simulink library "hcu_lib"  (R2021b)
settings: Solver=VariableStepAuto  StartTime=0.0  StopTime=10.0  RelTol=1e-3
undefined symbols (not defined in the file): ENUM_FAULTSTATE_FAIL, ENUM_FAULTSTATE_INDETERMINATE, ENUM_FAULTSTATE_PASS, EPSILON, FALSE, KPH2MPH, KPH2MPS, KXX2XX, MPH2KPH, MPS2KPH, ONE_INT16, ONE_INT32, RADPS2RPM, RPM2RADPS, slcm, TRUE, UNDEFINED_VALUE, XX2KXX, ZERO_FLOAT, ZERO_INT, ZERO_INT16, ZERO_INT32
libraries: $bdroot x31, simulink x10, afl x1
(part 1 of 3)
settings Model: Creator=12018  LastModifiedBy=FVT23010
settings SolverCC: AlgebraicLoopSolver=TrustRegion
settings DataIOCC: LimitDataPoints=on  SaveFormat=Array  SignalLoggingSaveFormat=ModelDataLogs  ReturnWorkspaceOutputs=off
settings OptimizationCC: BlockReduction=off  BooleanDataType=off  LifeSpan=inf
settings DebuggingCC: SaveWithParameterizedLinksMsg=none  UnderspecifiedInitializationDetection=Classic  MergeDetectMultiDrivingBlocksExec=none  SignalResolutionControl=TryResolveAllWithWarning  AllowSymbolicDim=off  SFUnexpectedBacktrackingDiag=warning  SFNoUnconditionalDefaultTransitionDiag=warning  SFExecutionAtInitializationDiag=none  SFMachineParentedDataDiag=warning  ArithmeticOperatorsInVariantConditions=warning
settings HardwareCC: TargetUnknown=on
settings ModelReferenceCC: PropagateSignalLabelsOutOfModel=off
settings SFSimCC: SimUseLocalCustomCode=off  CustomCodeUndefinedFunction=UseInterfaceOnly
settings RTWCC: RTWUseLocalCustomCode=off
settings CodeAppCC: StateflowObjectComments=on
settings GRTTargetCC: TargetLangStandard=C89/C90 (ANSI)
settings ConfigComp: CovMetricSettings=dw  CovSaveCumulativeToWorkspaceVar=on  CovSaveSingleToWorkspaceVar=on  CovExternalEMLEnable=off

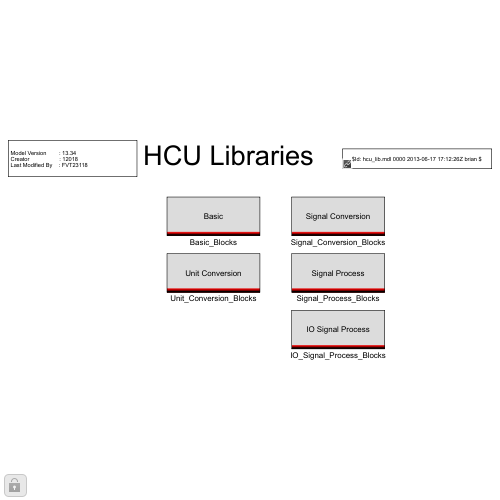
[thumbnail: Simulink's stored preview of the top-level diagram]
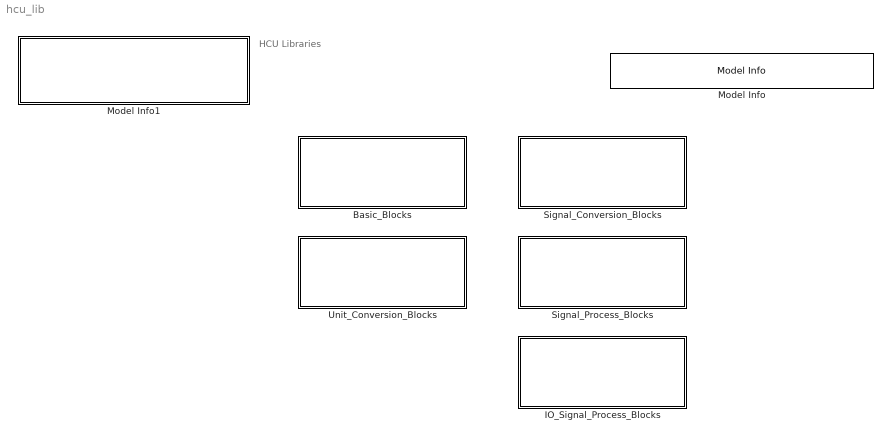
== system hcu_lib ==
  note: HCU Libraries
  Basic_Blocks : Subsystem
      mask Display:
      | patch([0 0 1 1], [0 1 1 0], [220/255 220/255 220/255]);
      | patch([0 0 1 1], [0 0.075 0.075 0], [230/255 0/255 0/255]);
      | patch([0 0 1 1], [0.025 0.05 0.05 0.025], [150/255 0/255 0/255]);
      | patch([0 0 1 1], [0 0.025 0.025 0], [0/255 0/255 0/255]);
      | 
      | disp('Basic')
  IO_Signal_Process_Blocks : Subsystem
      mask Display:
      | patch([0 0 1 1], [0 1 1 0], [220/255 220/255 220/255]);
      | patch([0 0 1 1], [0 0.075 0.075 0], [230/255 0/255 0/255]);
      | patch([0 0 1 1], [0.025 0.05 0.05 0.025], [150/255 0/255 0/255]);
      | patch([0 0 1 1], [0 0.025 0.025 0], [0/255 0/255 0/255]);
      | 
      | disp('IO Signal Process')
  Model Info : simulink/Model-Wide Utilities/Model Info  Frame=on  DisplayStringWithTags=$Id: hcu_lib.mdl 0000 2013-06-17 17:12:26Z brian $  HorizontalTextAlignment=Center  LeftAlignmentValue=0.5
  Model Info1 : Subsystem  LoadFcn=slcm LoadBlock;  InitFcn=slcm('UpdateAllCMBlocksInThisModelInit')  mask(CMBlock){InitialSaveTempField=, InitialBlockCM=, BlockCM=None, Frame=on, SaveTempField=, DisplayStringWithTags=|, MaskDisplayString=Model Version        : 13.85\nCreator                   : 12018\nLast Modified By    : FVT23010, HorizontalTextAlignment=Left, LeftAlignmentValue=0.02, SourceBlockDiagram=hcu_lib, TagMaxNumber=20, CMTag1=, CMTag2=, CMTag3=, CMTag4=, CMTag5=, CMTag6=, CMTag7=, CMTag8=, CMTag9=, CMTag10=, CMTag11=, CMTag12=, CMTag13=, CMTag14=, CMTag15=, CMTag16=, CMTag17=, CMTag18=, CMTag19=, CMTag20=}
      mask DisplayStringWithTags=|
      | Model Version        : %<ModelVersion>
      | Creator                   : %<Creator>
      | Last Modified By    : %<LastModifiedBy>
      mask help: This block allows revision control information to be displayed within the model.
      settings: CopyFcn=slcm CopyBlock;  DeleteFcn=slcm Cancel;  PostSaveFcn=slcm('UpdateAllCMBlocksInThisModel')  NameChangeFcn=slcm Rename;  OpenFcn=slcm
      mask Display: text(str2num(LeftAlignmentValue), 0.5, MaskDisplayString, 'HorizontalAlignment', HorizontalTextAlignment)
  Signal_Conversion_Blocks : Subsystem
      mask Display:
      | patch([0 0 1 1], [0 1 1 0], [220/255 220/255 220/255]);
      | patch([0 0 1 1], [0 0.075 0.075 0], [230/255 0/255 0/255]);
      | patch([0 0 1 1], [0.025 0.05 0.05 0.025], [150/255 0/255 0/255]);
      | patch([0 0 1 1], [0 0.025 0.025 0], [0/255 0/255 0/255]);
      | 
      | disp('Signal Conversion')
  Signal_Process_Blocks : Subsystem
      mask Display:
      | patch([0 0 1 1], [0 1 1 0], [220/255 220/255 220/255]);
      | patch([0 0 1 1], [0 0.075 0.075 0], [230/255 0/255 0/255]);
      | patch([0 0 1 1], [0.025 0.05 0.05 0.025], [150/255 0/255 0/255]);
      | patch([0 0 1 1], [0 0.025 0.025 0], [0/255 0/255 0/255]);
      | 
      | disp('Signal Process')
  Unit_Conversion_Blocks : Subsystem
      mask Display:
      | patch([0 0 1 1], [0 1 1 0], [220/255 220/255 220/255]);
      | patch([0 0 1 1], [0 0.075 0.075 0], [230/255 0/255 0/255]);
      | patch([0 0 1 1], [0.025 0.05 0.05 0.025], [150/255 0/255 0/255]);
      | patch([0 0 1 1], [0 0.025 0.025 0], [0/255 0/255 0/255]);
      | 
      | disp('Unit Conversion')

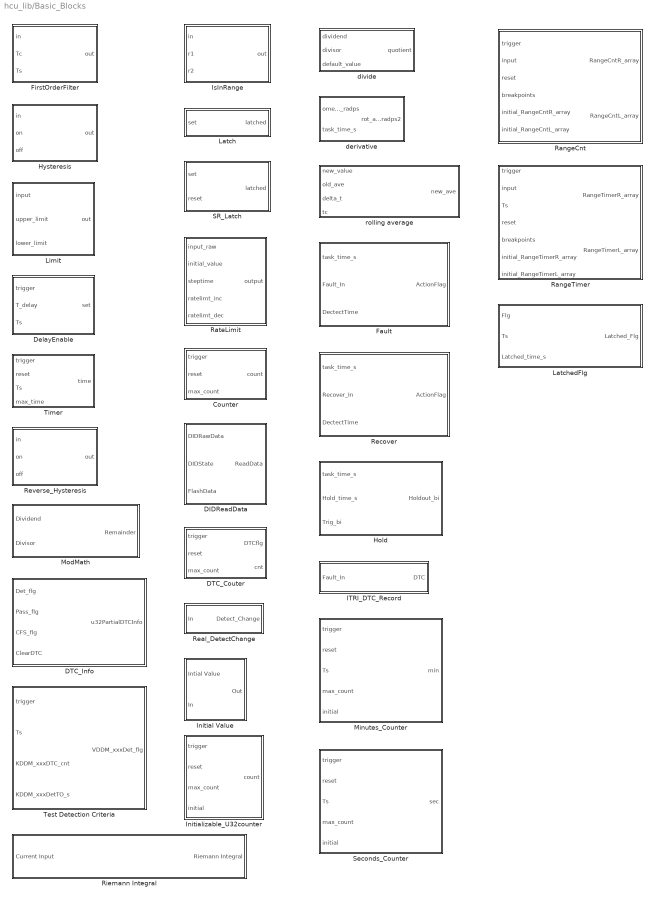
== system hcu_lib/Basic_Blocks ==
  Counter : Subsystem  mask(Count){}
      mask help: Counter function.
  DIDReadData : Subsystem  mask(Count){}
      mask help: Counter function.
  DTC_Couter : Subsystem  mask(Count){}
      mask help: Counter function.
  DTC_Info : Subsystem
  DelayEnable : Subsystem  mask(DelayEnable){}
      mask help: Delay enable funcion.
  Fault : Subsystem
  FirstOrderFilter : Subsystem  TreatAsAtomicUnit=on  RTWFileName=HCU_LIB  mask(FirstOrderFilter){}
      mask help: First order Filter.
      settings: RTWSystemCode=Inline  RTWFileNameOpts=User specified
  Hold : Subsystem
  Hysteresis : Subsystem  RTWFileName=HCU_LIB  mask(Hysteresis){}
      mask help: Hysteresis funcion.
      settings: RTWFileNameOpts=User specified
  ITRI_DTC_Record : Subsystem
  Initial Value : Subsystem  mask(Count){}
      mask help: Counter function.
  Initializable_U32counter : Subsystem  mask(Count){}
      mask help: Counter function.
  IsInRange : Subsystem  RTWFileName=HCU_LIB  mask(IsInRange){}
      mask help: Check the value range.
      settings: RTWFileNameOpts=User specified
  Latch : Subsystem  mask(Latch){}
      mask help: Latch function.
  LatchedFlg : Subsystem  mask(Latched Flg){}
      mask help: Latch flg function.
  Limit : Subsystem  RTWFileName=HCU_LIB  mask(Limit){}
      mask help: Limit funcion.
      settings: RTWFileNameOpts=User specified
  Minutes_Counter : Subsystem  mask(Min Count){}
      mask help: Minutes Counter.
  ModMath : Subsystem  mask(Count){}
      mask help: Counter function.
      mask Display:
      | fprintf('ModMath');
      | port_label('output', 1, 'Remainder');
      | port_label('input', 1, 'Dividend');
      | port_label('input', 2, 'Divisor');
  RangeCnt : Subsystem  mask(RangeCnt){}
      mask help: Range Counter.
  RangeTimer : Subsystem  mask(RangeTimer){}
      mask help: Range Timer (sec).
  RateLimit : Subsystem  RTWFileName=HCU_LIB  mask(RateLimit){}
      mask help: Rate limit function.
      settings: RTWFileNameOpts=User specified
  Real_DetectChange : Subsystem  mask(Count){}
      mask help: Counter function.
  Recover : Subsystem
  Reverse_Hysteresis : Subsystem  RTWFileName=HCU_LIB  mask(Hysteresis){}
      mask help: Hysteresis funcion.
      settings: RTWFileNameOpts=User specified
  Riemann Integral : Subsystem  mask(Riemann Integral){Ts=0.005, Total_T=1}
      mask prompts: Ts "Ts (s)"; Total_T "Total Time Interval (s)"
      mask help: Riemann Integral.
      mask Display:
      | fprintf('Ts (s): %4.3f \n Total Time Interval (s): %4.3f', Ts, Total_T);
      | 
      | port_label('input', 1, 'Current Input');
      | 
      | port_label('output', 1, ' Riemann Integral');
  SR_Latch : Subsystem  mask(SR_Latch){}
      mask help: SR latch function.
  Seconds_Counter : Subsystem  mask(Sec Count){}
      mask help: Seconds Counter.
  Test Detection Criteria : Subsystem
  Timer : Subsystem  mask(Timer){}
      mask help: Timer funcion.
  derivative : Subsystem  mask(Derative Block){}
      mask help: Simplified Derivative Calculation
      mask Display: disp(['Derivative'])
  divide : Subsystem  RTWFcnName=plaus_check  mask(divide){}
      mask help: Performs a division operation. If the divisor is found to be between -0.00001 and +0.00001 then a failsafe value is passed to the output.
      settings: RTWFcnNameOpts=User specified
      mask Display: disp('Divide');
  rolling average : Subsystem  RTWFcnName=rolav_tc  RTWFileName=HCU_LIB  mask(Rolling Average){}
      mask help:
      | Rolling Average - Time Constant.  This filter block is the first order approximation using a time constant.  Inputs include the time constant (entered through this dialogue), old_ave which is the previous average value, new_value which is the new filter to filter toward.
      |
      | The sample_interval which is elapsed time over which to perform the filter equation is computed internally - THIS BLOCK MUST BE CALLED EACH PASS to work as expected.
      settings: RTWFcnNameOpts=User specified  RTWFileNameOpts=User specified
      mask Display: disp('Rolling Average - TC')

== system hcu_lib/IO_Signal_Process_Blocks ==
  CAN_Msg_Validity_Process : Subsystem
  Protect : Subsystem  mask(Protect){}
      mask help: 2's complement calculation for protection function.
  RollCnt : Subsystem  mask(RollCnt){}
      mask help: Rolling counter function.
  RollCntValid : Subsystem  mask(RollCntValid){}
      mask help: Check valid signal of rolling counter signal.
  can_signal_process : Subsystem  mask(CANSignalProcess){}
      mask help: CAN signal process.
  digital_signal_process : Subsystem  mask(DigitalSignalProcess){}
      mask help: Digital signal process.
  hw_signal_process : Subsystem  mask(HWSignalProcess){}
      mask help: HW signal process.
  signal_out : Subsystem  mask(SignalOut){}
      mask help: Signal out.

== system hcu_lib/Model Info1 ==
  EmptySubsystem : Subsystem

== system hcu_lib/Signal_Conversion_Blocks ==
  Raw32 : Subsystem  mask(RawDataConversion){}
      mask help: Raw data conversion.
  conv_counts_to_eng_units : Subsystem  TreatAsAtomicUnit=on  RTWFcnName=unit_conversion  mask(Signal Conversion){}
      mask help: Converts counts to engineering units.
      settings: RTWSystemCode=Nonreusable function  RTWFcnNameOpts=User specified
  conv_eng_units_to_counts : Subsystem  TreatAsAtomicUnit=on  RTWFcnName=unit_conversion  mask(Signal Conversion){}
      mask help: Converts engineering units to counts.
      settings: RTWSystemCode=Nonreusable function  RTWFcnNameOpts=User specified
  convert_in : Subsystem  mask(ConvertIn){gain=UNDEFINED_VALUE, offset=UNDEFINED_VALUE}
      mask help:
      | Conversion Formula
      |
      | The conversion formula is
      |
      | raw_value = (physical_value - Offset) / Factor
      |
      | where physical_value is the value of the signal after it is saturated using the specified Min and Max values. raw_value is the packed signal value.
  convert_out : Subsystem  mask(ConvertOut){gain=UNDEFINED_VALUE, offset=UNDEFINED_VALUE}
      mask help:
      | Conversion Formula
      |
      | The conversion formula is
      |
      | raw_value = (physical_value - Offset) / Factor
      |
      | where physical_value is the value of the signal after it is saturated using the specified Min and Max values. raw_value is the packed signal value.

== system hcu_lib/Signal_Process_Blocks ==
  fault_filter_latch : Subsystem  TreatAsAtomicUnit=on  RTWFcnName=ff_latch  RTWFileName=HCU_LIB  mask(FaultFilterLatch){}
      mask help: Fault filter latch.
      settings: RTWFcnNameOpts=Use subsystem name  RTWFileNameOpts=User specified
  fault_filter_reset : Subsystem  TreatAsAtomicUnit=on  RTWFcnName=ff_reset  RTWFileName=HCU_LIB  mask(FaultFilterReset){}
      mask help: Fault filter reset.
      settings: RTWSystemCode=Inline  RTWFcnNameOpts=Use subsystem name  RTWFileNameOpts=User specified
  latching fault filter reinit : Subsystem  TreatAsAtomicUnit=on  RTWFcnName=ff_latching  RTWFileName=HCU_LIB  mask(Latching Fault Filter){}
      mask help: Fault filter block - Latches the fault output flag to TRUE if the input flag is repeatedly set True.
      settings: RTWFcnNameOpts=User specified  RTWFileNameOpts=User specified
      mask Display: disp('Latching\nFault Filter')
  latching_fault_filter : Subsystem  TreatAsAtomicUnit=on  RTWFcnName=ff_latching  RTWFileName=HCU_LIB  mask(Latching Fault Filter){}
      mask help: Fault filter block - Latches the fault output flag to TRUE if the input flag is repeatedly set True.
      settings: RTWFcnNameOpts=Use subsystem name  RTWFileNameOpts=User specified
      mask Display: disp('Latching\nFault Filter')
  override_signal_m1 : Subsystem  TreatAsAtomicUnit=on  RTWFcnName=srvc_ovrd  RTWFileName=HCU_LIB  mask(Override Function){}
      mask help: Override funcion for signal.
      settings: RTWFcnNameOpts=Use subsystem name  RTWFileNameOpts=User specified
  "override_signal_m2 " : Subsystem  TreatAsAtomicUnit=on  RTWFcnName=srvc_ovrd  RTWFileName=HCU_LIB  mask(Override Function with Service){}
      mask help: Override function with service for signal.
      settings: RTWFcnNameOpts=Use subsystem name  RTWFileNameOpts=User specified
  sig_valid_check : Subsystem  TreatAsAtomicUnit=on  RTWFcnName=sig_valid_check  RTWFileName=HCU_LIB  mask(SignalValidCheck){}
      mask help: Signal valid check.
      settings: RTWFcnNameOpts=User specified  RTWFileNameOpts=User specified

== system hcu_lib/Unit_Conversion_Blocks ==
  km2miles : Subsystem  mask(Conversion){}
      mask help: Convert kilometers to miles.
      mask Display: disp('km \rightarrow mile', 'texmode', 'on')
  kph2mps : Subsystem  mask(Conversion){}
      mask help: Convert Kilometers per hour to Meters per second
      mask Display: disp('km/h \rightarrow m/s', 'texmode', 'on')
  kxx2xx : Subsystem  mask(Conversion){}
      mask help: Multiply by 1000.
      mask Display: disp('kiloxx \rightarrow xx', 'texmode', 'on')
  litres2gallons : Subsystem  mask(Conversion){UK=off}
      mask prompts: UK "UK Gallon"
      mask help: Convert litres to gallons.
      mask Display: disp('litre \rightarrow gallon', 'texmode', 'on')
  miles2km : Subsystem  mask(Conversion){}
      mask help: Convert kilometers to miles.
      mask Display: disp('mile \rightarrow km', 'texmode', 'on')
  mps2kph : Subsystem  mask(Conversion){}
      mask help: Convert Meters per second to Kilometers per hour
      mask Display: disp('m/s \rightarrow km/h', 'texmode', 'on')
  radps2rpm : Subsystem
      mask help: Converst radians per second to revolutions per minute.
      mask Display: disp('rad/s \rightarrow rpm', 'texmode', 'on')
  rpm2radps : Subsystem
      mask help: Converts revolutions per minute to radians per second.
      mask Display: disp('rpm \rightarrow rad/s', 'texmode', 'on')
  xx2kxx : Subsystem  mask(Conversion){}
      mask help: Divides by 1000.
      mask Display: disp('xx \rightarrow kiloxx', 'texmode', 'on')

== system hcu_lib/Basic_Blocks/Counter ==
  note: /* Max Value of counter is 65535 */
  trigger : Inport
  reset : Inport  Port=2
  max_count : Inport  Port=3
  Constant1 : Constant  Value=ZERO_INT16  OutDataTypeStr=uint16
  Constant2 : Constant  Value=uint16(1)  OutDataTypeStr=single
  MinMax : MinMax  Inputs=2
  Saturation : Saturate  UpperLimit=65535  LowerLimit=0
      settings: AttributesFormatString=<upper = %<UpperLimit>>\n<lower = %<LowerLimit>>
  Subtract2 : Sum
  Switch1 : Switch  Criteria=u2 ~= 0
      settings: AttributesFormatString=<%<Criteria>>
  Switch2 : Switch  Criteria=u2 ~= 0
      settings: AttributesFormatString=<%<Criteria>>
  Unit Delay1 : UnitDelay  SampleTime=-1  HasFrameUpgradeWarning=on
      settings: AttributesFormatString=<initial = %<X0>>
  count : Outport
  wires:
  Saturation/1 -> MinMax/1
  [last_count] -> Subtract2/1
  max_count/1 -> Saturation/1
  Unit Delay1/1 -> Switch2/3, [last_count]
  MinMax/1 -> count/1, Unit Delay1/1
  Constant2/1 -> Subtract2/2
  Constant1/1 -> Switch1/1
  reset/1 -> Switch1/2
  Subtract2/1 -> Switch2/1
  Switch1/1 -> MinMax/2
  Switch2/1 -> Switch1/3
  trigger/1 -> Switch2/2

== system hcu_lib/Basic_Blocks/DIDReadData ==
  DIDRawData : Inport
  DIDState : Inport  Port=2
  FlashData : Inport  Port=3
  Constant9 : Constant  Value=FALSE
  Data Type Conversion : DataTypeConversion  OutDataTypeStr=boolean
  Data Type Conversion1 : DataTypeConversion  OutDataTypeStr=uint8
  Data Type Conversion2 : DataTypeConversion  OutDataTypeStr=uint8
  Equal4 : RelationalOperator  Operator===  OutDataTypeStr=boolean  RndMeth=Simplest
  Latch1 : Subsystem  mask(Latch){}
      mask help: Latch function.
  Switch4 : Switch  Criteria=u2 ~= 0
  Switch5 : Switch  Criteria=u2 ~= 0
  Unit Delay2 : UnitDelay  SampleTime=-1  HasFrameUpgradeWarning=on
  ReadData : Outport
  wires:
  Constant9/1 -> Equal4/2
  [LastReadData] -> Switch5/3
  Equal4/1 -> Latch1/1(set), Switch5/2
  DIDState/1 -> Data Type Conversion/1
  Latch1/1(latched) -> Switch4/2
  Switch5/1 -> Switch4/1
  Switch4/1 -> Data Type Conversion1/1
  DIDRawData/1 -> Switch5/1
  FlashData/1 -> Switch4/3
  Data Type Conversion/1 -> Equal4/1
  Data Type Conversion1/1 -> ReadData/1, Unit Delay2/1
  Unit Delay2/1 -> Data Type Conversion2/1
  Data Type Conversion2/1 -> [LastReadData]

== system hcu_lib/Basic_Blocks/DTC_Couter ==
  note: /* Max Value of counter is 255 */
  trigger : Inport
  reset : Inport  Port=2
  max_count : Inport  Port=3
  Constant1 : Constant  Value=ZERO_INT
  Constant2 : Constant  Value=uint8(1)  OutDataTypeStr=uint8
  MinMax : MinMax  Inputs=2
  Relational Operator : RelationalOperator  OutDataTypeStr=boolean  RndMeth=Simplest
  Saturation : Saturate  UpperLimit=255  LowerLimit=0
      settings: AttributesFormatString=<upper = %<UpperLimit>>\n<lower = %<LowerLimit>>
  Subtract2 : Sum
  Switch1 : Switch  Criteria=u2 ~= 0
      settings: AttributesFormatString=<%<Criteria>>
  Switch2 : Switch  Criteria=u2 ~= 0
      settings: AttributesFormatString=<%<Criteria>>
  Unit Delay1 : UnitDelay  SampleTime=-1  HasFrameUpgradeWarning=on
      settings: AttributesFormatString=<initial = %<X0>>
  DTCflg : Outport
  cnt : Outport  Port=2
  wires:
  trigger/1 -> Switch2/2
  Switch2/1 -> Switch1/3
  Switch1/1 -> MinMax/2
  Subtract2/1 -> Switch2/1
  reset/1 -> Switch1/2
  Constant1/1 -> Switch1/1
  Constant2/1 -> Subtract2/2
  MinMax/1 -> Unit Delay1/1, Relational Operator/1, cnt/1
  Unit Delay1/1 -> [last_count], Switch2/3
  max_count/1 -> Saturation/1
  [last_count] -> Subtract2/1
  Saturation/1 -> [max_count], MinMax/1
  [max_count] -> Relational Operator/2
  Relational Operator/1 -> DTCflg/1

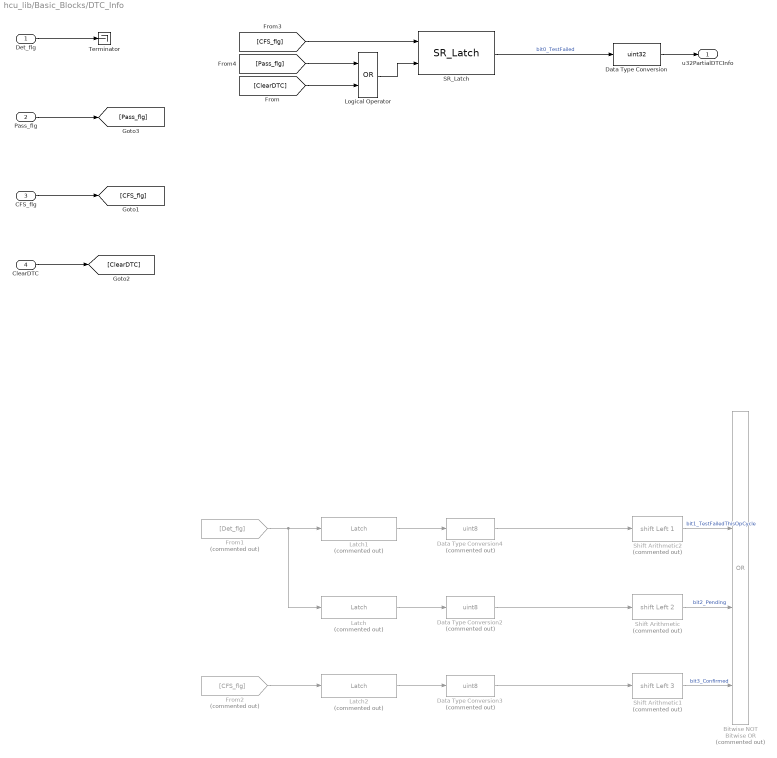
== system hcu_lib/Basic_Blocks/DTC_Info ==
  Det_flg : Inport
  Pass_flg : Inport  Port=2
  CFS_flg : Inport  Port=3
  ClearDTC : Inport  Port=4
  Bitwise NOT : simulink/Logic and Bit Operations/Bitwise Operator  Commented=on  logicop=OR  UseBitMask=off  NumInputPorts=4  BitMask=bin2dec('11011001')  BitMaskRealWorld=Stored Integer
  Data Type Conversion : DataTypeConversion  OutDataTypeStr=uint32
  Data Type Conversion2 : DataTypeConversion  Commented=on  OutDataTypeStr=uint8
  Data Type Conversion3 : DataTypeConversion  Commented=on  OutDataTypeStr=uint8
  Data Type Conversion4 : DataTypeConversion  Commented=on  OutDataTypeStr=uint8
  From1 : From  Commented=on  GotoTag=Det_flg
  From2 : From  Commented=on  GotoTag=CFS_flg
  Latch : $bdroot/Basic_Blocks/Latch  Commented=on
  Latch1 : $bdroot/Basic_Blocks/Latch  Commented=on
  Latch2 : $bdroot/Basic_Blocks/Latch  Commented=on
  Logical Operator : Logic  Operator=OR  AllPortsSameDT=off  OutDataTypeStr=boolean
  SR_Latch : $bdroot/Basic_Blocks/SR_Latch
  Shift Arithmetic : ArithShift  Commented=on  BitShiftNumber=2  BitShiftDirection=Left
  Shift Arithmetic1 : ArithShift  Commented=on  BitShiftNumber=3  BitShiftDirection=Left
  Shift Arithmetic2 : ArithShift  Commented=on  BitShiftNumber=1  BitShiftDirection=Left
  Terminator : Terminator
  u32PartialDTCInfo : Outport
  wires:
  SR_Latch/1 -> Data Type Conversion/1  "bit0_TestFailed"
  Data Type Conversion2/1 -> Shift Arithmetic/1
  Data Type Conversion3/1 -> Shift Arithmetic1/1
  Data Type Conversion/1 -> u32PartialDTCInfo/1
  Det_flg/1 -> Terminator/1
  [CFS_flg] -> SR_Latch/1
  From1/1 -> Latch1/1, Latch/1
  Latch1/1 -> Data Type Conversion4/1
  Data Type Conversion4/1 -> Shift Arithmetic2/1
  CFS_flg/1 -> [CFS_flg]
  From2/1 -> Latch2/1
  Pass_flg/1 -> [Pass_flg]
  [Pass_flg] -> Logical Operator/1
  Latch2/1 -> Data Type Conversion3/1
  Latch/1 -> Data Type Conversion2/1
  Shift Arithmetic2/1 -> Bitwise NOT/2  "bit1_TestFailedThisOpCycle"
  Shift Arithmetic/1 -> Bitwise NOT/3  "bit2_Pending"
  Shift Arithmetic1/1 -> Bitwise NOT/4  "bit3_Confirmed"
  ClearDTC/1 -> [ClearDTC]
  [ClearDTC] -> Logical Operator/2
  Logical Operator/1 -> SR_Latch/2

== system hcu_lib/Basic_Blocks/DelayEnable ==
  trigger : Inport
  T_delay : Inport  Port=2
  Ts : Inport  Port=3
  Constant1 : Constant  Value=ZERO_FLOAT
  Constant2 : Constant  Value=ZERO_FLOAT
  Relational Operator1 : RelationalOperator  Operator=>  OutDataTypeStr=boolean  RndMeth=Nearest
  Subtract1 : Sum
  Switch : Switch  Criteria=u2 ~= 0
      settings: AttributesFormatString=<%<Criteria>>
  Switch1 : Switch  Criteria=u2 ~= 0
      settings: AttributesFormatString=<%<Criteria>>
  Unit Delay : UnitDelay  SampleTime=-1  HasFrameUpgradeWarning=on
      settings: AttributesFormatString=<intial = %<X0>>
  Unit Delay1 : UnitDelay  InitialCondition=FALSE  SampleTime=-1  HasFrameUpgradeWarning=on
      settings: AttributesFormatString=<intial = %<X0>>
  set : Outport
  wires:
  Unit Delay1/1 -> Switch1/2
  Constant2/1 -> Switch1/1
  Ts/1 -> Switch1/3
  Switch1/1 -> Subtract1/2
  Unit Delay/1 -> Subtract1/1
  Relational Operator1/1 -> Unit Delay1/1, set/1
  trigger/1 -> Switch/2
  T_delay/1 -> Relational Operator1/2
  Constant1/1 -> Switch/3
  Switch/1 -> Unit Delay/1, Relational Operator1/1
  Subtract1/1 -> Switch/1

== system hcu_lib/Basic_Blocks/Fault ==
  task_time_s : Inport
  Fault_In : Inport  Port=2
  DectectTime : Inport  Port=3
  AND : Logic  AllPortsSameDT=off  OutDataTypeStr=boolean
  Add1 : Sum
  Constant62 : Constant  Value=ZERO_FLOAT
  NOT : Logic  Operator=NOT  AllPortsSameDT=off  OutDataTypeStr=boolean
  Relational Operator2 : RelationalOperator  OutDataTypeStr=boolean  RndMeth=Simplest
  Switch6 : Switch  Criteria=u2 > Threshold
  Unit Delay1 : UnitDelay  SampleTime=-1  HasFrameUpgradeWarning=on
  Unit Delay2 : UnitDelay  SampleTime=-1  HasFrameUpgradeWarning=on
  ActionFlag : Outport
  wires:
  Relational Operator2/1 -> Unit Delay1/1, ActionFlag/1
  Constant62/1 -> Switch6/3
  Add1/1 -> Switch6/1
  Fault_In/1 -> AND/1
  Unit Delay2/1 -> Add1/1
  DectectTime/1 -> Relational Operator2/2
  task_time_s/1 -> Add1/2
  Switch6/1 -> Unit Delay2/1, Relational Operator2/1
  Unit Delay1/1 -> NOT/1
  AND/1 -> Switch6/2
  NOT/1 -> AND/2

== system hcu_lib/Basic_Blocks/FirstOrderFilter ==
  in : Inport
  Tc : Inport  Port=2
  Ts : Inport  Port=3
  Add : Sum
  Add2 : Sum  Inputs=+-
  Constant3 : Constant  OutDataTypeStr=single
  Constant4 : Constant  Value=0  OutDataTypeStr=single
  Constant5 : Constant  Value=0  OutDataTypeStr=single
  Constant6 : Constant  Value=eps  OutDataTypeStr=single
  Divide : Product  Inputs=*/
  MinMax{1..4} (4 alike) : MinMax  Function=max  Inputs=2
  Product : Product  RndMeth=Zero
  Product1 : Product  RndMeth=Zero
  Unit Delay : UnitDelay  SampleTime=-1  HasFrameUpgradeWarning=on
  out : Outport
  wires:
  Add/1 -> out/1, Unit Delay/1
  Divide/1 -> Product1/1, Add2/2
  Constant3/1 -> Add2/1
  Add2/1 -> Product/2
  Product/1 -> Add/1
  Unit Delay/1 -> Product/1
  in/1 -> Product1/2
  Product1/1 -> Add/2
  Tc/1 -> MinMax2/1
  Constant4/1 -> MinMax2/2
  Ts/1 -> MinMax3/1
  Constant5/1 -> MinMax3/2
  MinMax3/1 -> MinMax1/2
  MinMax2/1 -> Divide/1, MinMax1/1
  MinMax1/1 -> MinMax4/1
  Constant6/1 -> MinMax4/2
  MinMax4/1 -> Divide/2

== system hcu_lib/Basic_Blocks/Hold ==
  task_time_s : Inport
  Hold_time_s : Inport  Port=2
  Trig_bi : Inport  Port=3
  Add1 : Sum
  Constant62 : Constant  Value=ZERO_FLOAT
  Detect Decrease : simulink/Logic and Bit Operations/Detect Decrease  vinit=0.0  OutDataTypeStr=boolean
  OR : Logic  Operator=OR  AllPortsSameDT=off  OutDataTypeStr=boolean
  Relational Operator2 : RelationalOperator  OutDataTypeStr=boolean  RndMeth=Simplest
  SR_Latch : $bdroot/Basic_Blocks/SR_Latch
  Switch6 : Switch  Criteria=u2 > Threshold
  Unit Delay1 : UnitDelay  SampleTime=-1  HasFrameUpgradeWarning=on
  Unit Delay2 : UnitDelay  SampleTime=-1  HasFrameUpgradeWarning=on
  Holdout_bi : Outport
  wires:
  Switch6/1 -> Relational Operator2/1, Unit Delay2/1
  task_time_s/1 -> Add1/2
  Hold_time_s/1 -> Relational Operator2/2
  Unit Delay2/1 -> Add1/1
  Add1/1 -> Switch6/1
  Constant62/1 -> Switch6/3
  Relational Operator2/1 -> Unit Delay1/1
  Trig_bi/1 -> OR/2, Detect Decrease/1
  SR_Latch/1 -> Switch6/2, OR/1
  Detect Decrease/1 -> SR_Latch/1
  Unit Delay1/1 -> SR_Latch/2
  OR/1 -> Holdout_bi/1

== system hcu_lib/Basic_Blocks/Hysteresis ==
  in : Inport
  on : Inport  Port=2
  off : Inport  Port=3
  Logical Operator1 : Logic  AllPortsSameDT=off  OutDataTypeStr=boolean
  Logical Operator2 : Logic  AllPortsSameDT=off  OutDataTypeStr=boolean
  Logical Operator3 : Logic  Operator=NOT  AllPortsSameDT=off  OutDataTypeStr=boolean
  RESET : Constant  Value=0  OutDataTypeStr=boolean
  Relational Operator1 : RelationalOperator  OutDataTypeStr=boolean  RndMeth=Nearest
  Relational Operator2 : RelationalOperator  Operator=<  OutDataTypeStr=boolean  RndMeth=Nearest
  SET : Constant  OutDataTypeStr=boolean
  Switch : Switch  Criteria=u2 ~= 0
  Switch1 : Switch  Criteria=u2 ~= 0
  Unit Delay : UnitDelay  SampleTime=-1  HasFrameUpgradeWarning=on
  out : Outport
  wires:
  in/1 -> Relational Operator1/1, Relational Operator2/1
  on/1 -> Relational Operator1/2
  off/1 -> Relational Operator2/2
  Relational Operator1/1 -> Logical Operator1/1
  Relational Operator2/1 -> Logical Operator2/1
  Logical Operator1/1 -> Switch/2
  SET/1 -> Switch/1
  Switch/1 -> Switch1/3
  Logical Operator2/1 -> Switch1/2
  RESET/1 -> Switch1/1
  Switch1/1 -> out/1, Unit Delay/1
  Unit Delay/1 -> Switch/3, Logical Operator3/1, Logical Operator2/2
  Logical Operator3/1 -> Logical Operator1/2

== system hcu_lib/Basic_Blocks/ITRI_DTC_Record ==
  Fault_In : Inport
  Event Status Enum : Subsystem  mask{EventStatusEnum=[0, 1, 2, 3], EventStatusIndex=FAILED}
      mask prompts: EventStatusEnum "Enum"; EventStatusIndex "Event Status"
      mask TypeOptions EventStatusIndex: PASSED | FAILED | PRE-PASSED | PRE-FAILED
      mask Display: map = ["PASSED", "FAILED", "PRE-PASSED", "PRE-FAILED"];disp("" + map(EventStatusIndex) + ": " + EventStatusEnum(EventStatusIndex));
  Event Status Enum1 : $bdroot/Basic_Blocks/ITRI_DTC_Record/Event Status Enum  EventStatusEnum=[0, 1, 2, 3]  EventStatusIndex=PASSED
  Switch : Switch  Criteria=u2 > Threshold
  DTC : Outport
  wires:
  Fault_In/1 -> Switch/2
  Event Status Enum/1(Event Status) -> Switch/1
  Event Status Enum1/1 -> Switch/3
  Switch/1 -> DTC/1

== system hcu_lib/Basic_Blocks/Initial Value ==
  Intial Value : Inport
  In : Inport  Port=2
  Constant : Constant  Value=TRUE
  Switch : Switch  Criteria=u2 > Threshold
  Unit Delay : UnitDelay  SampleTime=-1  HasFrameUpgradeWarning=on
  Out : Outport
  wires:
  Switch/1 -> Out/1
  Constant/1 -> Unit Delay/1
  Unit Delay/1 -> Switch/2
  In/1 -> Switch/1
  Intial Value/1 -> Switch/3

== system hcu_lib/Basic_Blocks/Initializable_U32counter ==
  note: /* Max Value of counter is 65535 */
  trigger : Inport
  reset : Inport  Port=2
  max_count : Inport  Port=3
  initial : Inport  Port=4
  Constant1 : Constant  Value=ZERO_INT32  OutDataTypeStr=uint16
  Constant2 : Constant  Value=ONE_INT32  OutDataTypeStr=uint32
  Initial Value : $bdroot/Basic_Blocks/Initial Value
  MinMax : MinMax  Inputs=2
  Saturation : Saturate  UpperLimit=65535  LowerLimit=0
      settings: AttributesFormatString=<upper = %<UpperLimit>>\n<lower = %<LowerLimit>>
  Subtract2 : Sum
  Switch1 : Switch  Criteria=u2 ~= 0
      settings: AttributesFormatString=<%<Criteria>>
  Switch2 : Switch  Criteria=u2 ~= 0
      settings: AttributesFormatString=<%<Criteria>>
  Unit Delay1 : UnitDelay  SampleTime=-1  HasFrameUpgradeWarning=on
      settings: AttributesFormatString=<initial = %<X0>>
  count : Outport
  wires:
  trigger/1 -> Switch2/2
  Switch2/1 -> Switch1/3
  Switch1/1 -> MinMax/2
  Subtract2/1 -> Switch2/1
  reset/1 -> Switch1/2
  Constant1/1 -> Switch1/1
  Constant2/1 -> Subtract2/2
  MinMax/1 -> Unit Delay1/1, count/1
  max_count/1 -> Saturation/1
  Saturation/1 -> MinMax/1
  Unit Delay1/1 -> Initial Value/2
  Initial Value/1 -> [last_count]
  [last_count] -> Switch2/3
  [last_count] -> Subtract2/1
  initial/1 -> Initial Value/1

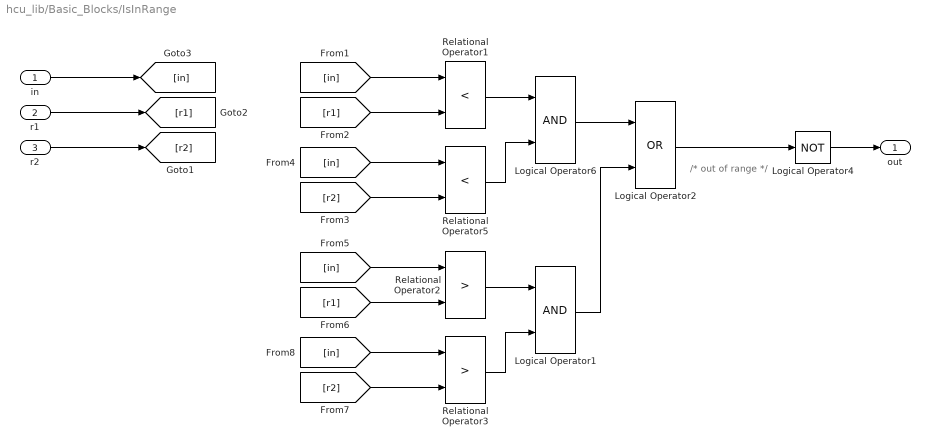
== system hcu_lib/Basic_Blocks/IsInRange ==
  note: /* out of range */
  in : Inport
  r1 : Inport  Port=2
  r2 : Inport  Port=3
  Logical Operator1 : Logic  AllPortsSameDT=off  OutDataTypeStr=boolean
  Logical Operator2 : Logic  Operator=OR  AllPortsSameDT=off  OutDataTypeStr=boolean
  Logical Operator4 : Logic  Operator=NOT  AllPortsSameDT=off  OutDataTypeStr=boolean
  Logical Operator6 : Logic  AllPortsSameDT=off  OutDataTypeStr=boolean
  Relational Operator1 : RelationalOperator  Operator=<  OutDataTypeStr=boolean  RndMeth=Nearest
  Relational Operator2 : RelationalOperator  Operator=>  OutDataTypeStr=boolean  RndMeth=Nearest
  Relational Operator3 : RelationalOperator  Operator=>  OutDataTypeStr=boolean  RndMeth=Nearest
  Relational Operator5 : RelationalOperator  Operator=<  OutDataTypeStr=boolean  RndMeth=Nearest
  out : Outport
  wires:
  Relational Operator1/1 -> Logical Operator6/1
  Relational Operator5/1 -> Logical Operator6/2
  Logical Operator6/1 -> Logical Operator2/1
  in/1 -> [in]
  r1/1 -> [r1]
  r2/1 -> [r2]
  [in] -> Relational Operator1/1
  [r1] -> Relational Operator1/2
  [in] -> Relational Operator5/1
  [r2] -> Relational Operator5/2
  Relational Operator2/1 -> Logical Operator1/1
  Relational Operator3/1 -> Logical Operator1/2
  [in] -> Relational Operator2/1
  [r1] -> Relational Operator2/2
  [in] -> Relational Operator3/1
  [r2] -> Relational Operator3/2
  Logical Operator1/1 -> Logical Operator2/2
  Logical Operator2/1 -> Logical Operator4/1
  Logical Operator4/1 -> out/1

== system hcu_lib/Basic_Blocks/Latch ==
  set : Inport
  Data Type Conversion : DataTypeConversion  OutDataTypeStr=boolean
  Switch1 : Switch  Criteria=u2 ~= 0  Threshold=0.5
      settings: AttributesFormatString=<Criteria=%<Criteria>>
  Unit Delay : UnitDelay  SampleTime=-1  HasFrameUpgradeWarning=on
  latched : Outport
  wires:
  Unit Delay/1 -> Switch1/1, Data Type Conversion/1
  Switch1/1 -> Unit Delay/1, latched/1
  set/1 -> Switch1/3
  Data Type Conversion/1 -> Switch1/2

== system hcu_lib/Basic_Blocks/LatchedFlg ==
  Flg : Inport
  Ts : Inport  Port=2
  Latched_time_s : Inport  Port=3
  AND1 : Logic  Operator=OR  AllPortsSameDT=off  OutDataTypeStr=boolean
  AND2 : Logic  AllPortsSameDT=off  OutDataTypeStr=boolean
  AND3 : Logic  AllPortsSameDT=off  OutDataTypeStr=boolean
  Equal1 : RelationalOperator  OutDataTypeStr=boolean  RndMeth=Simplest
  NOT : Logic  Operator=NOT  AllPortsSameDT=off  OutDataTypeStr=boolean
  NOT1 : Logic  Operator=NOT  AllPortsSameDT=off  OutDataTypeStr=boolean
  SR_Latch : $bdroot/Basic_Blocks/SR_Latch
  Timer : $bdroot/Basic_Blocks/Timer
  Unit Delay : UnitDelay  SampleTime=-1  HasFrameUpgradeWarning=on
  Unit Delay2 : UnitDelay  SampleTime=-1  HasFrameUpgradeWarning=on
  Latched_Flg : Outport
  wires:
  Flg/1 -> AND1/1, NOT/1, SR_Latch/1
  AND1/1 -> Timer/2, NOT1/1
  [Reset] -> Unit Delay/1
  [Reset] -> Unit Delay2/1
  Timer/1 -> Equal1/1
  Equal1/1 -> [Reset]
  Unit Delay2/1 -> AND1/2
  SR_Latch/1 -> Latched_Flg/1, AND3/1
  Ts/1 -> Timer/3
  Latched_time_s/1 -> [Latched_time_s]
  [Latched_time_s] -> Timer/4
  [Latched_time_s] -> Equal1/2
  AND2/1 -> SR_Latch/2
  Unit Delay/1 -> AND2/2
  NOT/1 -> AND2/1
  AND3/1 -> Timer/1
  NOT1/1 -> AND3/2

== system hcu_lib/Basic_Blocks/Limit ==
  input : Inport
  upper_limit : Inport  Port=2
  lower_limit : Inport  Port=3
  MinMax10 : MinMax  Function=max  Inputs=2
  MinMax5 : MinMax  Inputs=2
  out : Outport
  wires:
  lower_limit/1 -> MinMax10/2
  upper_limit/1 -> MinMax5/2
  MinMax10/1 -> out/1
  input/1 -> MinMax5/1
  MinMax5/1 -> MinMax10/1

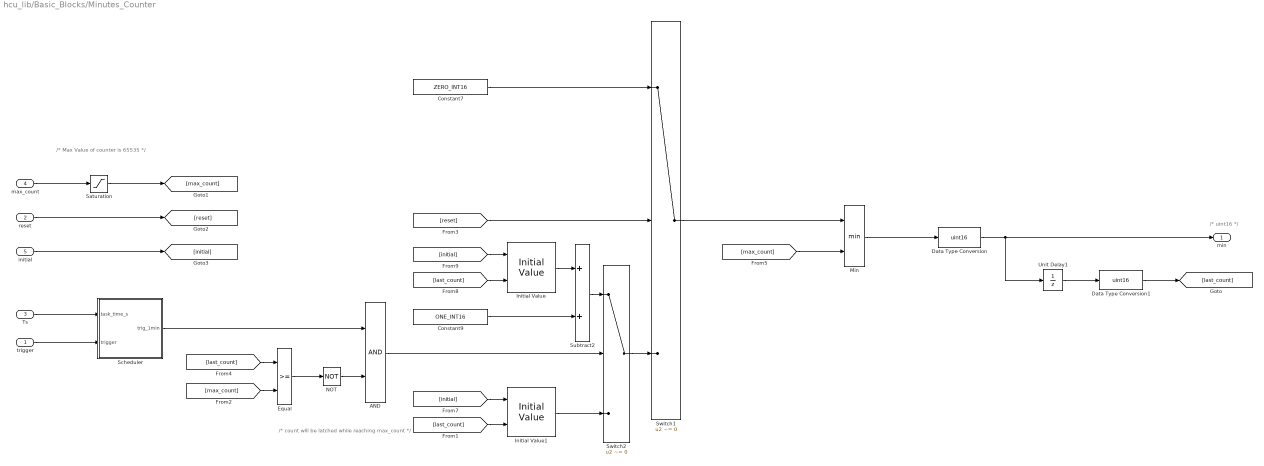
== system hcu_lib/Basic_Blocks/Minutes_Counter ==
  note: /* uint16 */
  note: /* Max Value of counter is 65535 */
  note: /* count will be latched while reaching max_count */
  trigger : Inport
  reset : Inport  Port=2
  Ts : Inport  Port=3
  max_count : Inport  Port=4
  initial : Inport  Port=5
  AND : Logic  AllPortsSameDT=off  OutDataTypeStr=boolean
  Constant7 : Constant  Value=ZERO_INT16  OutDataTypeStr=uint16
  Constant9 : Constant  Value=ONE_INT16  OutDataTypeStr=single
  Data Type Conversion : DataTypeConversion  OutDataTypeStr=uint16
  Data Type Conversion1 : DataTypeConversion  OutDataTypeStr=uint16
  Equal : RelationalOperator  OutDataTypeStr=boolean  RndMeth=Simplest
  Initial Value : $bdroot/Basic_Blocks/Initial Value
  Initial Value1 : $bdroot/Basic_Blocks/Initial Value
  Min : MinMax  Inputs=2
  NOT : Logic  Operator=NOT  AllPortsSameDT=off  OutDataTypeStr=boolean
  Saturation : Saturate  UpperLimit=65535  LowerLimit=0
      settings: AttributesFormatString=<upper = %<UpperLimit>>\n<lower = %<LowerLimit>>
  Scheduler : Stateflow chart  TreatAsAtomicUnit=on
  Subtract2 : Sum
  Switch1 : Switch  Criteria=u2 ~= 0
      settings: AttributesFormatString=<%<Criteria>>
  Switch2 : Switch  Criteria=u2 ~= 0
      settings: AttributesFormatString=<%<Criteria>>
  Unit Delay1 : UnitDelay  SampleTime=-1  HasFrameUpgradeWarning=on
      settings: AttributesFormatString=<initial = %<X0>>
  min : Outport
  wires:
  Data Type Conversion1/1 -> [last_count]
  max_count/1 -> Saturation/1
  reset/1 -> [reset]
  Unit Delay1/1 -> Data Type Conversion1/1
  Data Type Conversion/1 -> min/1, Unit Delay1/1
  Min/1 -> Data Type Conversion/1
  [max_count] -> Equal/2
  NOT/1 -> AND/2
  [last_count] -> Equal/1
  Switch1/1 -> Min/1
  Saturation/1 -> [max_count]
  Scheduler/1(trig_1min) -> AND/1
  Equal/1 -> NOT/1
  [max_count] -> Min/2
  Ts/1 -> Scheduler/1(task_time_s)
  trigger/1 -> Scheduler/2(trigger)
  initial/1 -> [initial]
  [last_count] -> Initial Value1/2
  Initial Value1/1 -> Switch2/3
  [initial] -> Initial Value1/1
  Switch2/1 -> Switch1/3
  Subtract2/1 -> Switch2/1
  [last_count] -> Initial Value/2
  [reset] -> Switch1/2
  Constant9/1 -> Subtract2/2
  AND/1 -> Switch2/2
  [initial] -> Initial Value/1
  Initial Value/1 -> Subtract2/1
  Constant7/1 -> Switch1/1

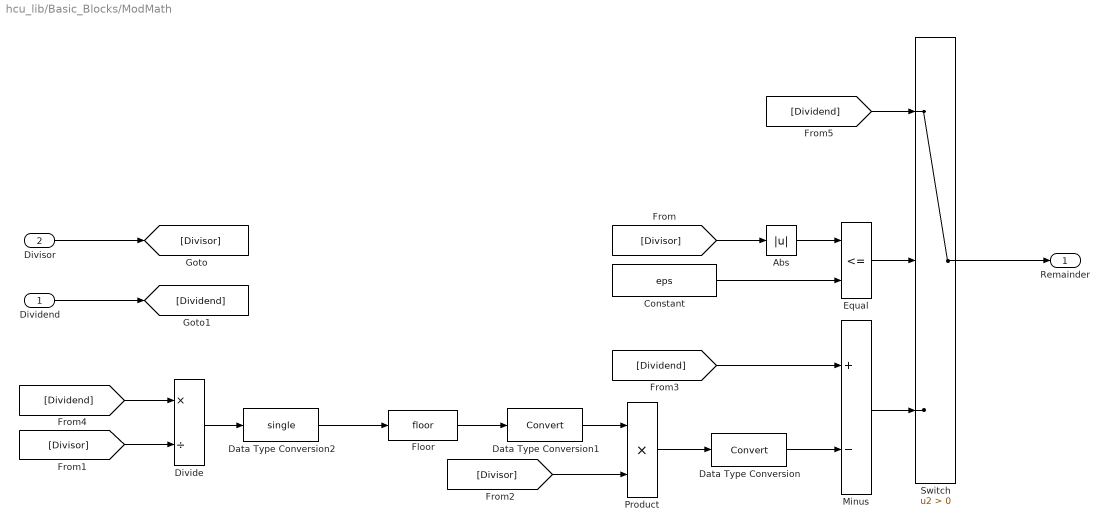
== system hcu_lib/Basic_Blocks/ModMath ==
  Dividend : Inport
  Divisor : Inport  Port=2
  Abs : Abs
  Constant : Constant  Value=eps
  Data Type Conversion : DataTypeConversion
  Data Type Conversion1 : DataTypeConversion
  Data Type Conversion2 : DataTypeConversion  OutDataTypeStr=single
  Divide : Product  Inputs=*/
  Equal : RelationalOperator  Operator=<=  OutDataTypeStr=boolean  RndMeth=Simplest
  Floor : Rounding
  Minus : Sum  Inputs=+-
  Product : Product
  Switch : Switch  Criteria=u2 > Threshold
  Remainder : Outport
  wires:
  Divisor/1 -> [Divisor]
  Equal/1 -> Switch/2
  Constant/1 -> Equal/2
  [Dividend] -> Divide/1
  Switch/1 -> Remainder/1
  [Dividend] -> Switch/1
  Minus/1 -> Switch/3
  Data Type Conversion2/1 -> Floor/1
  Data Type Conversion/1 -> Minus/2
  [Dividend] -> Minus/1
  Dividend/1 -> [Dividend]
  Floor/1 -> Data Type Conversion1/1
  Data Type Conversion1/1 -> Product/1
  [Divisor] -> Divide/2
  Abs/1 -> Equal/1
  [Divisor] -> Product/2
  Divide/1 -> Data Type Conversion2/1
  Product/1 -> Data Type Conversion/1
  [Divisor] -> Abs/1

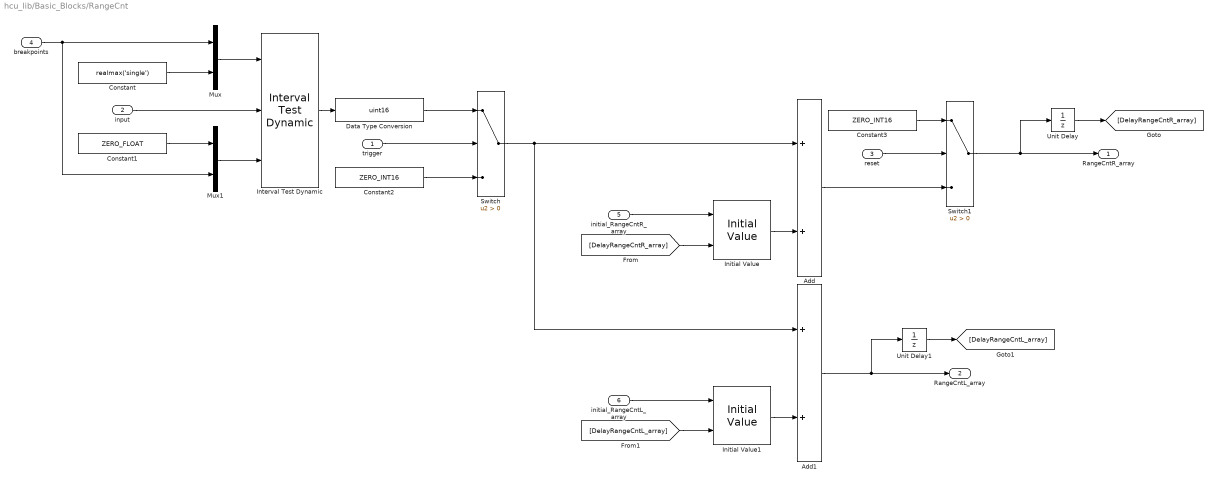
== system hcu_lib/Basic_Blocks/RangeCnt ==
  trigger : Inport
  input : Inport  Port=2
  reset : Inport  Port=3
  breakpoints : Inport  Port=4
  initial_RangeCntR_array : Inport  Port=5
  initial_RangeCntL_array : Inport  Port=6
  Add : Sum
  Add1 : Sum
  Constant : Constant  Value=realmax('single')
  Constant1 : Constant  Value=ZERO_FLOAT
  Constant2 : Constant  Value=ZERO_INT16
  Constant3 : Constant  Value=ZERO_INT16
  Data Type Conversion : DataTypeConversion  OutDataTypeStr=uint16
  Initial Value : $bdroot/Basic_Blocks/Initial Value
  Initial Value1 : $bdroot/Basic_Blocks/Initial Value
  Interval Test Dynamic : simulink/Logic and Bit Operations/Interval Test Dynamic  IntervalClosedRight=off  IntervalClosedLeft=on  OutDataTypeStr=boolean
      settings: SourceProductBaseCode=SL
  Mux : Mux  Inputs=2
  Mux1 : Mux  Inputs=2
  Switch : Switch  Criteria=u2 > Threshold
  Switch1 : Switch  Criteria=u2 > Threshold
  Unit Delay : UnitDelay  SampleTime=-1  HasFrameUpgradeWarning=on
  Unit Delay1 : UnitDelay  SampleTime=-1  HasFrameUpgradeWarning=on
  RangeCntR_array : Outport
  RangeCntL_array : Outport  Port=2
  wires:
  breakpoints/1 -> Mux1/2, Mux/1
  Constant3/1 -> Switch1/1
  Switch1/1 -> Unit Delay/1, RangeCntR_array/1
  Add/1 -> Switch1/3
  reset/1 -> Switch1/2
  Initial Value/1 -> Add/2
  [DelayRangeCntR_array] -> Initial Value/2
  input/1 -> Interval Test Dynamic/2
  initial_RangeCntR_array/1 -> Initial Value/1
  Constant1/1 -> Mux1/1
  trigger/1 -> Switch/2
  Unit Delay/1 -> [DelayRangeCntR_array]
  Switch/1 -> Add1/1, Add/1
  Constant/1 -> Mux/2
  Mux1/1 -> Interval Test Dynamic/3
  Constant2/1 -> Switch/3
  Mux/1 -> Interval Test Dynamic/1
  initial_RangeCntL_array/1 -> Initial Value1/1
  [DelayRangeCntL_array] -> Initial Value1/2
  Initial Value1/1 -> Add1/2
  Add1/1 -> Unit Delay1/1, RangeCntL_array/1
  Unit Delay1/1 -> [DelayRangeCntL_array]
  Interval Test Dynamic/1 -> Data Type Conversion/1
  Data Type Conversion/1 -> Switch/1

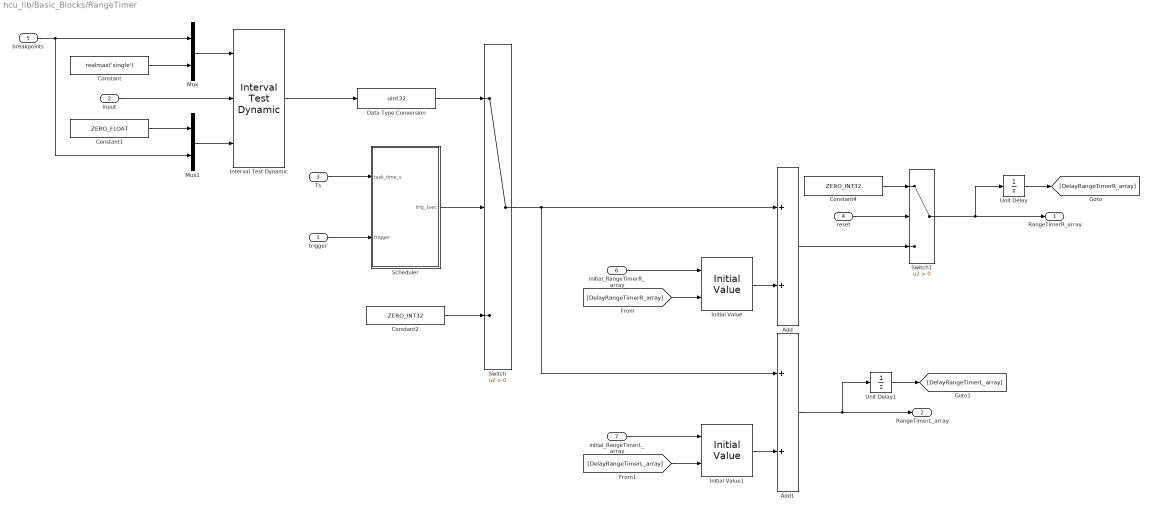
== system hcu_lib/Basic_Blocks/RangeTimer ==
  trigger : Inport
  input : Inport  Port=2
  Ts : Inport  Port=3
  reset : Inport  Port=4
  breakpoints : Inport  Port=5
  initial_RangeTimerR_array : Inport  Port=6
  initial_RangeTimerL_array : Inport  Port=7
  Add : Sum
  Add1 : Sum
  Constant : Constant  Value=realmax('single')
  Constant1 : Constant  Value=ZERO_FLOAT
  Constant2 : Constant  Value=ZERO_INT32
  Constant4 : Constant  Value=ZERO_INT32
  Data Type Conversion : DataTypeConversion  OutDataTypeStr=uint32
  Initial Value : $bdroot/Basic_Blocks/Initial Value
  Initial Value1 : $bdroot/Basic_Blocks/Initial Value
  Interval Test Dynamic : simulink/Logic and Bit Operations/Interval Test Dynamic  IntervalClosedRight=off  IntervalClosedLeft=on  OutDataTypeStr=boolean
      settings: SourceProductBaseCode=SL
  Mux : Mux  Inputs=2
  Mux1 : Mux  Inputs=2
  Scheduler : Stateflow chart  TreatAsAtomicUnit=on
  Switch : Switch  Criteria=u2 > Threshold
  Switch1 : Switch  Criteria=u2 > Threshold
  Unit Delay : UnitDelay  SampleTime=-1  HasFrameUpgradeWarning=on
  Unit Delay1 : UnitDelay  SampleTime=-1  HasFrameUpgradeWarning=on
  RangeTimerR_array : Outport
  RangeTimerL_array : Outport  Port=2
  wires:
  Data Type Conversion/1 -> Switch/1
  Interval Test Dynamic/1 -> Data Type Conversion/1
  Unit Delay1/1 -> [DelayRangeTimerL_array]
  Add1/1 -> RangeTimerL_array/1, Unit Delay1/1
  Initial Value1/1 -> Add1/2
  [DelayRangeTimerL_array] -> Initial Value1/2
  initial_RangeTimerL_array/1 -> Initial Value1/1
  Mux/1 -> Interval Test Dynamic/1
  Constant2/1 -> Switch/3
  Mux1/1 -> Interval Test Dynamic/3
  Constant/1 -> Mux/2
  Switch/1 -> Add/1, Add1/1
  Unit Delay/1 -> [DelayRangeTimerR_array]
  Constant1/1 -> Mux1/1
  initial_RangeTimerR_array/1 -> Initial Value/1
  input/1 -> Interval Test Dynamic/2
  [DelayRangeTimerR_array] -> Initial Value/2
  Initial Value/1 -> Add/2
  reset/1 -> Switch1/2
  Add/1 -> Switch1/3
  Switch1/1 -> RangeTimerR_array/1, Unit Delay/1
  Constant4/1 -> Switch1/1
  breakpoints/1 -> Mux/1, Mux1/2
  trigger/1 -> Scheduler/2(trigger)
  Ts/1 -> Scheduler/1(task_time_s)
  Scheduler/1(trig_1sec) -> Switch/2

== system hcu_lib/Basic_Blocks/RateLimit ==
  input_raw : Inport
  initial_value : Inport  Port=2
  steptime : Inport  Port=3
  ratelimt_inc : Inport  Port=4
  ratelimt_dec : Inport  Port=5
  MinMax : MinMax  Inputs=2
  MinMax1 : MinMax  Function=max  Inputs=2
  MinMax2 : MinMax  Function=max  Inputs=2
  MinMax3 : MinMax  Inputs=2
  Product : Product  RndMeth=Zero
  Product1 : Product  RndMeth=Zero
  Resettable Delay : Delay  DelayLength=1  InitialConditionSource=Input port
      settings: InputPortMap=u0,p4
  Sum5 : Sum  Inputs=+-
  Sum6 : Sum
  step_time6 : Constant  Value=0  OutDataTypeStr=single
  output : Outport
  wires:
  ratelimt_dec/1 -> Product1/2
  steptime/1 -> Product1/1, Product/2
  Sum5/1 -> MinMax1/1
  [Dec] -> MinMax1/2
  [Inc] -> MinMax/1
  MinMax1/1 -> MinMax/2
  MinMax/1 -> Sum6/1
  input_raw/1 -> Sum5/1
  Sum6/1 -> Resettable Delay/1, output/1
  Resettable Delay/1 -> Sum5/2, Sum6/2
  Product/1 -> MinMax2/1
  Product1/1 -> MinMax3/2
  step_time6/1 -> MinMax2/2, MinMax3/1
  MinMax2/1 -> [Inc]
  MinMax3/1 -> [Dec]
  ratelimt_inc/1 -> Product/1
  initial_value/1 -> Resettable Delay/2

== system hcu_lib/Basic_Blocks/Real_DetectChange ==
  In : Inport
  Constant : Constant  Value=TRUE
  Detect Change : simulink/Logic and Bit Operations/Detect Change  vinit=0  OutDataTypeStr=boolean
  Logical Operator : Logic  AllPortsSameDT=off  OutDataTypeStr=boolean
  Unit Delay : UnitDelay  SampleTime=-1  HasFrameUpgradeWarning=on
  Detect_Change : Outport
  wires:
  Unit Delay/1 -> Logical Operator/2
  Constant/1 -> Unit Delay/1
  In/1 -> Detect Change/1
  Detect Change/1 -> Logical Operator/1
  Logical Operator/1 -> Detect_Change/1

== system hcu_lib/Basic_Blocks/Recover ==
  task_time_s : Inport
  Recover_In : Inport  Port=2
  DectectTime : Inport  Port=3
  AND : Logic  AllPortsSameDT=off  OutDataTypeStr=boolean
  Add1 : Sum
  Constant62 : Constant  Value=ZERO_FLOAT
  NOT : Logic  Operator=NOT  AllPortsSameDT=off  OutDataTypeStr=boolean
  Relational Operator2 : RelationalOperator  OutDataTypeStr=boolean  RndMeth=Simplest
  Switch6 : Switch  Criteria=u2 > Threshold
  Unit Delay1 : UnitDelay  SampleTime=-1  HasFrameUpgradeWarning=on
  Unit Delay2 : UnitDelay  SampleTime=-1  HasFrameUpgradeWarning=on
  ActionFlag : Outport
  wires:
  NOT/1 -> AND/2
  AND/1 -> Switch6/2
  Unit Delay1/1 -> NOT/1
  Switch6/1 -> Relational Operator2/1, Unit Delay2/1
  task_time_s/1 -> Add1/2
  DectectTime/1 -> Relational Operator2/2
  Unit Delay2/1 -> Add1/1
  Recover_In/1 -> AND/1
  Add1/1 -> Switch6/1
  Constant62/1 -> Switch6/3
  Relational Operator2/1 -> ActionFlag/1, Unit Delay1/1

== system hcu_lib/Basic_Blocks/Reverse_Hysteresis ==
  in : Inport
  on : Inport  Port=2
  off : Inport  Port=3
  Logical Operator1 : Logic  AllPortsSameDT=off  OutDataTypeStr=boolean
  Logical Operator2 : Logic  AllPortsSameDT=off  OutDataTypeStr=boolean
  Logical Operator3 : Logic  Operator=NOT  AllPortsSameDT=off  OutDataTypeStr=boolean
  RESET : Constant  Value=0  OutDataTypeStr=boolean
  Relational Operator1 : RelationalOperator  Operator=<=  OutDataTypeStr=boolean  RndMeth=Nearest
  Relational Operator2 : RelationalOperator  Operator=>  OutDataTypeStr=boolean  RndMeth=Nearest
  SET : Constant  OutDataTypeStr=boolean
  Switch : Switch  Criteria=u2 ~= 0
  Switch1 : Switch  Criteria=u2 ~= 0
  Unit Delay : UnitDelay  SampleTime=-1  HasFrameUpgradeWarning=on
  out : Outport
  wires:
  Logical Operator3/1 -> Logical Operator1/2
  Unit Delay/1 -> Logical Operator2/2, Logical Operator3/1, Switch/3
  Switch1/1 -> Unit Delay/1, out/1
  RESET/1 -> Switch1/1
  Logical Operator2/1 -> Switch1/2
  Switch/1 -> Switch1/3
  SET/1 -> Switch/1
  Logical Operator1/1 -> Switch/2
  Relational Operator2/1 -> Logical Operator2/1
  Relational Operator1/1 -> Logical Operator1/1
  off/1 -> Relational Operator2/2
  on/1 -> Relational Operator1/2
  in/1 -> Relational Operator2/1, Relational Operator1/1

== system hcu_lib/Basic_Blocks/Riemann Integral ==
  Current Input : Inport
  Constant : Constant  Value=Ts  OutDataTypeStr=single
  Delay : Delay  DelayLength=Total_T/Ts  DelayLengthUpperLimit=1000
  Minus : Sum  Inputs=+-
  Minus1 : Sum
  Product : Product
  Unit Delay : UnitDelay  SampleTime=-1  HasFrameUpgradeWarning=on
  " Riemann Integral" : Outport
  wires:
  Current Input/1 -> Delay/1, Minus/1
  Minus1/1 -> Unit Delay/1, " Riemann Integral"/1
  Delay/1 -> Minus/2
  Product/1 -> Minus1/1
  Minus/1 -> Product/1
  Constant/1 -> Product/2
  Unit Delay/1 -> Minus1/2

== system hcu_lib/Basic_Blocks/SR_Latch ==
  set : Inport
  reset : Inport  Port=2
  Data Type Conversion : DataTypeConversion  OutDataTypeStr=boolean
  Logical Operator : Logic  AllPortsSameDT=off  OutDataTypeStr=boolean
  Logical Operator1 : Logic  Operator=NOT  AllPortsSameDT=off  OutDataTypeStr=boolean
  Switch1 : Switch  Criteria=u2 ~= 0  Threshold=0.5
      settings: AttributesFormatString=<Criteria=%<Criteria>>
  Switch2 : Switch  Criteria=u2 ~= 0  Threshold=0.5
      settings: AttributesFormatString=<Criteria=%<Criteria>>
  Unit Delay : UnitDelay  SampleTime=-1  HasFrameUpgradeWarning=on
  latched : Outport
  wires:
  Logical Operator1/1 -> Switch2/1, Logical Operator/2
  Logical Operator/1 -> Switch1/2
  Switch2/1 -> Switch1/3
  Unit Delay/1 -> Switch2/3
  reset/1 -> Logical Operator1/1, Switch2/2
  set/1 -> Logical Operator/1, Switch1/1
  Switch1/1 -> Data Type Conversion/1
  Data Type Conversion/1 -> latched/1, Unit Delay/1

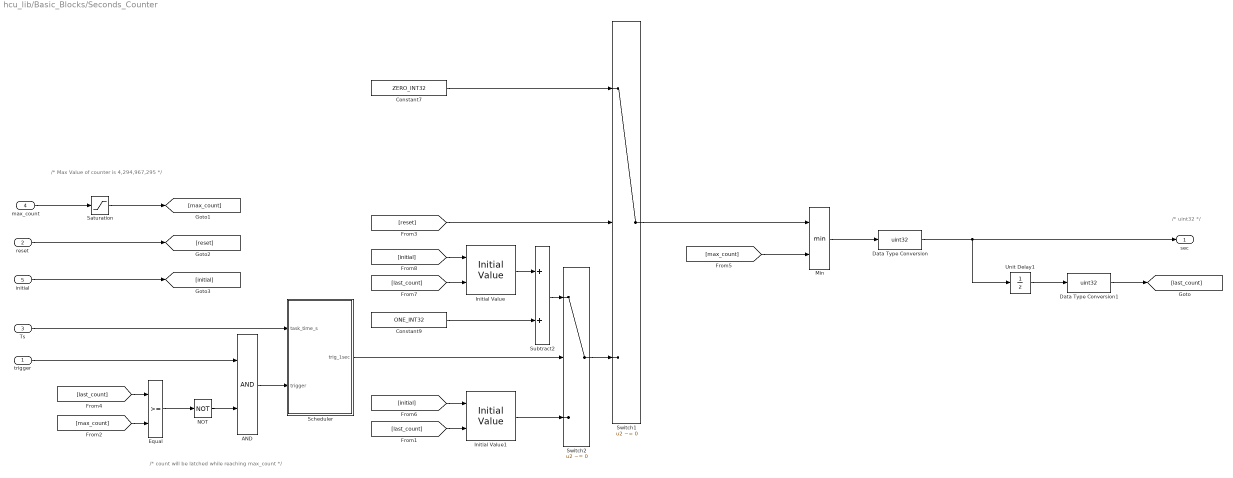
== system hcu_lib/Basic_Blocks/Seconds_Counter ==
  note: /* count will be latched while reaching max_count */
  note: /* uint32 */
  note: /* Max Value of counter is 4,294,967,295 */
  trigger : Inport
  reset : Inport  Port=2
  Ts : Inport  Port=3
  max_count : Inport  Port=4
  initial : Inport  Port=5
  AND : Logic  AllPortsSameDT=off  OutDataTypeStr=boolean
  Constant7 : Constant  Value=ZERO_INT32  OutDataTypeStr=uint16
  Constant9 : Constant  Value=ONE_INT32  OutDataTypeStr=single
  Data Type Conversion : DataTypeConversion  OutDataTypeStr=uint32
  Data Type Conversion1 : DataTypeConversion  OutDataTypeStr=uint32
  Equal : RelationalOperator  OutDataTypeStr=boolean  RndMeth=Simplest
  Initial Value : $bdroot/Basic_Blocks/Initial Value
  Initial Value1 : $bdroot/Basic_Blocks/Initial Value
  Min : MinMax  Inputs=2
  NOT : Logic  Operator=NOT  AllPortsSameDT=off  OutDataTypeStr=boolean
  Saturation : Saturate  UpperLimit=4294967295  LowerLimit=0
      settings: AttributesFormatString=<upper = %<UpperLimit>>\n<lower = %<LowerLimit>>
  Scheduler : Stateflow chart  TreatAsAtomicUnit=on
  Subtract2 : Sum
  Switch1 : Switch  Criteria=u2 ~= 0
      settings: AttributesFormatString=<%<Criteria>>
  Switch2 : Switch  Criteria=u2 ~= 0
      settings: AttributesFormatString=<%<Criteria>>
  Unit Delay1 : UnitDelay  SampleTime=-1  HasFrameUpgradeWarning=on
      settings: AttributesFormatString=<initial = %<X0>>
  sec : Outport
  wires:
  Data Type Conversion1/1 -> [last_count]
  Unit Delay1/1 -> Data Type Conversion1/1
  Data Type Conversion/1 -> Unit Delay1/1, sec/1
  Ts/1 -> Scheduler/1(task_time_s)
  Subtract2/1 -> Switch2/1
  Constant9/1 -> Subtract2/2
  Switch2/1 -> Switch1/3
  Constant7/1 -> Switch1/1
  max_count/1 -> Saturation/1
  Scheduler/1(trig_1sec) -> Switch2/2
  reset/1 -> [reset]
  [reset] -> Switch1/2
  Equal/1 -> NOT/1
  AND/1 -> Scheduler/2(trigger)
  trigger/1 -> AND/1
  NOT/1 -> AND/2
  [last_count] -> Equal/1
  Saturation/1 -> [max_count]
  [max_count] -> Equal/2
  [max_count] -> Min/2
  Min/1 -> Data Type Conversion/1
  Switch1/1 -> Min/1
  initial/1 -> [initial]
  Initial Value1/1 -> Switch2/3
  [last_count] -> Initial Value1/2
  [initial] -> Initial Value1/1
  Initial Value/1 -> Subtract2/1
  [initial] -> Initial Value/1
  [last_count] -> Initial Value/2

== system hcu_lib/Basic_Blocks/Test Detection Criteria ==
  trigger : Inport
  Ts : Inport  Port=2
  KDDM_xxxDTC_cnt : Inport  Port=3
  KDDM_xxxDetTO_s : Inport  Port=4
  Constant35 : Constant  Value=ZERO_INT
  Data Type Conversion : DataTypeConversion  OutDataTypeStr=single
  Data Type Conversion1 : DataTypeConversion  OutDataTypeStr=uint16
  Detect Increase : simulink/Logic and Bit Operations/Detect Increase  vinit=0.0  OutDataTypeStr=boolean
  Equal9 : RelationalOperator  Operator===  OutDataTypeStr=boolean  RndMeth=Simplest
  Gain : Gain  Gain=KXX2XX  RndMeth=Round
  Gain1 : Gain  Gain=KXX2XX
  Logical Operator19 : Logic  AllPortsSameDT=off  OutDataTypeStr=boolean
  Logical Operator3 : Logic  Operator=NOT  AllPortsSameDT=off  OutDataTypeStr=boolean
  ModMath : Subsystem  mask(Count){}
      mask help: Counter function.
      mask Display:
      | fprintf('ModMath');
      | port_label('output', 1, 'Remainder');
      | port_label('input', 1, 'Dividend');
      | port_label('input', 2, 'Divisor');
  Product : Product
  Rounding Function : Rounding  Operator=round
  Rounding Function1 : Rounding  Operator=round
  Timer : Subsystem  mask(Timer){}
      mask help: Timer funcion.
  VDDM_xxxDet_flg : Outport
  wires:
  Constant35/1 -> Equal9/2
  Logical Operator19/1 -> Detect Increase/1
  trigger/1 -> Timer/1(trigger), Logical Operator19/1, Logical Operator3/1
  [KDDM_xxxDetTO_s] -> Gain1/1
  Equal9/1 -> Logical Operator19/2
  Logical Operator3/1 -> Timer/2(reset)
  Timer/1(time) -> Gain/1
  Ts/1 -> Timer/3(Ts)
  Product/1 -> Timer/4(max_time)
  Data Type Conversion/1 -> Product/2
  KDDM_xxxDetTO_s/1 -> [KDDM_xxxDetTO_s], Product/1
  KDDM_xxxDTC_cnt/1 -> Data Type Conversion/1
  ModMath/1(Remainder) -> Data Type Conversion1/1
  Detect Increase/1 -> VDDM_xxxDet_flg/1
  Gain/1 -> Rounding Function/1
  Gain1/1 -> Rounding Function1/1
  Data Type Conversion1/1 -> Equal9/1
  Rounding Function/1 -> ModMath/1(Dividend)
  Rounding Function1/1 -> ModMath/2(Divisor)
